simulink library "ExampleModel_lib"  (Simulink 7.9)
settings: Solver=ode45  StartTime=0.0  StopTime=10.0  RelTol=1e-3
libraries: powerlib x11, powerlib_extras x4, ExampleModel_lib x1
settings Model: RequirementInfo="{}  %GIDa_6317c1c3_1285_46a1_a401_c249d430af69"  Creator=jde1  LastModifiedBy=jde1

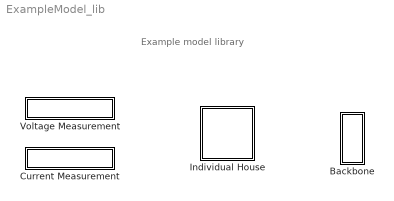
== system ExampleModel_lib ==
  note: Example model library
  Backbone : Subsystem  mask{length=0.0465}
  Current Measurement : Subsystem  StopFcn=|
      | myname = getfullname(gcb);                                                                      
      | rto = get_param([myname '/RMS Display'], 'RuntimeObject');                                      
      | set_param(myname, 'MaskDisplay', ['color(''blue''); disp(' num2str(rto.InputPort(1).Data) ')']);
      mask Display:
      | port_label('lconn', 1, '+')
      | port_label('rconn', 1, '-')
      | color('blue')
      | disp('0')
  Individual House : Subsystem  mask{length=0.02}
      mask prompts: length "Length of service line"
      mask Display:
      | plot([20 30 40 20 20 40 40], [30 40 30 30 10 10 30])
      | port_label('LConn',1,'+')
      | port_label('RConn',1,'-')
  Voltage Measurement : Subsystem  StopFcn=|
      | myname = getfullname(gcb);                                                                      
      | rto = get_param([myname '/RMS Display'], 'RuntimeObject');                                      
      | set_param(myname, 'MaskDisplay', ['color(''blue''); disp(' num2str(rto.InputPort(1).Data) ')']);
      mask Display:
      | port_label('lconn', 1, '+')
      | port_label('rconn', 1, '-')
      | color('blue')
      | disp('0')

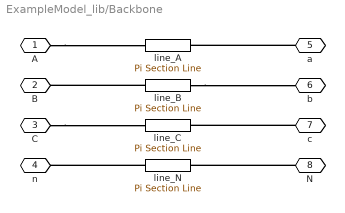
== system ExampleModel_lib/Backbone ==
  line_A : powerlib/Elements/Pi Section Line  LConnTagsString=__new0  RConnTagsString=__new0  Frequency=50  Resistance=0.497  Inductance=1.2032e-3  Capacitance=1e-9  Length=length  PiSections=1  Measurements=None
      settings: AttributesFormatString=\n
  line_B : powerlib/Elements/Pi Section Line  LConnTagsString=__new0  RConnTagsString=__new0  Frequency=50  Resistance=0.497  Inductance=1.2032e-3  Capacitance=1e-9  Length=length  PiSections=1  Measurements=None
      settings: AttributesFormatString=\n
  line_C : powerlib/Elements/Pi Section Line  LConnTagsString=__new0  RConnTagsString=__new0  Frequency=50  Resistance=0.497  Inductance=1.2032e-3  Capacitance=1e-9  Length=length  PiSections=1  Measurements=None
      settings: AttributesFormatString=\n
  line_N : powerlib/Elements/Pi Section Line  LConnTagsString=__new0  RConnTagsString=__new0  Frequency=50  Resistance=0.497  Inductance=1.2032e-3  Capacitance=1e-9  Length=length  PiSections=1  Measurements=None
      settings: AttributesFormatString=\n
  A : PMIOPort  Port=1  Side=Left
  B : PMIOPort  Port=2  Side=Left
  C : PMIOPort  Port=3  Side=Left
  n : PMIOPort  Port=4  Side=Left
  a : PMIOPort  Port=5  Side=Right
  b : PMIOPort  Port=6  Side=Right
  c : PMIOPort  Port=7  Side=Right
  N : PMIOPort  Port=8  Side=Right
  connections:
  line_N/RConn1 -- n/RConn1
  N/RConn1 -- line_N/LConn1
  a/RConn1 -- line_A/RConn1
  line_B/RConn1 -- b/RConn1
  c/RConn1 -- line_C/RConn1
  C/RConn1 -- line_C/LConn1
  line_B/LConn1 -- B/RConn1
  A/RConn1 -- line_A/LConn1

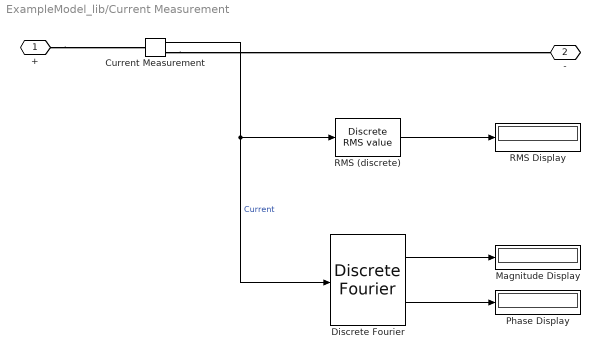
== system ExampleModel_lib/Current Measurement ==
  Current Measurement : powerlib/Measurements/Current Measurement  PhasorSimulation=off  OutputType=Complex  PSBequivalent=0
  Discrete Fourier : powerlib_extras/Discrete Measurements/Discrete  Fourier  Freq=50  n=1  Par_Init=[0 0]  Ts=0.001
  Magnitude Display : Display
  Phase Display : Display
  RMS (discrete) : powerlib_extras/Discrete Measurements/Discrete  RMS value  Freq=50  Mag_Init=0  Ts=0.001
  RMS Display : Display
  + : PMIOPort  Port=1  Side=Left
  - : PMIOPort  Port=2  Side=Right
  wires:
  RMS (discrete)/1 -> RMS Display/1
  Discrete Fourier/1 -> Magnitude Display/1
  Discrete Fourier/2 -> Phase Display/1
  Current Measurement/1 -> Discrete Fourier/1, RMS (discrete)/1  "Current"
  connections:
  +/RConn1 -- Current Measurement/LConn1
  Current Measurement/RConn1 -- -/RConn1

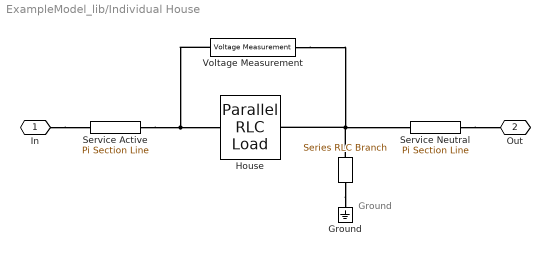
== system ExampleModel_lib/Individual House ==
  note: Ground
  " " : powerlib/Elements/Series RLC Branch  LConnTagsString=__new0  RConnTagsString=__new0  BranchType=R  Resistance=10  Inductance=1e-3  SetiL0=off  InitialCurrent=0  Capacitance=1e-6  Setx0=off  InitialVoltage=0  Measurements=None
  Ground : powerlib/Elements/Ground  LConnTagsString=a
  House : powerlib/Elements/Parallel RLC Load  LConnTagsString=a  RConnTagsString=__new0  NominalVoltage=230  NominalFrequency=50  ActivePower=500  InductivePower=1  CapacitivePower=1  Setx0=off  InitialVoltage=0  SetiL0=off  InitialCurrent=0  Measurements=None
      settings: AttributesFormatString=\n
  Service Active : powerlib/Elements/Pi Section Line  LConnTagsString=__new0  RConnTagsString=__new0  Frequency=50  Resistance=2.33  Inductance=2.833e-4  Capacitance=1e-9  Length=length  PiSections=1  Measurements=None
      settings: AttributesFormatString=\n
  Service Neutral : powerlib/Elements/Pi Section Line  LConnTagsString=__new0  RConnTagsString=__new0  Frequency=50  Resistance=2.33  Inductance=2.833e-4  Capacitance=1e-9  Length=length  PiSections=1  Measurements=None
      settings: AttributesFormatString=\n
  Voltage Measurement : ExampleModel_lib/Voltage Measurement  SystemSampleTime=-1
  In : PMIOPort  Port=1  Side=Left
  Out : PMIOPort  Port=2  Side=Right
  connections:
  Voltage Measurement/LConn1 -- House/LConn1 -- Service Active/RConn1
  " "/RConn1 -- Ground/LConn1
  " "/LConn1 -- House/RConn1 -- Voltage Measurement/RConn1 -- Service Neutral/LConn1
  In/RConn1 -- Service Active/LConn1
  Service Neutral/RConn1 -- Out/RConn1

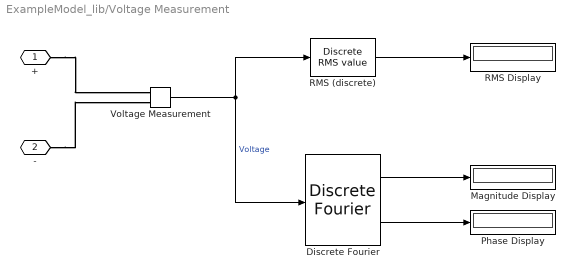
== system ExampleModel_lib/Voltage Measurement ==
  Discrete Fourier : powerlib_extras/Discrete Measurements/Discrete  Fourier  Freq=50  n=1  Par_Init=[0 0]  Ts=0.001
  Magnitude Display : Display
  Phase Display : Display
  RMS (discrete) : powerlib_extras/Discrete Measurements/Discrete  RMS value  Freq=50  Mag_Init=0  Ts=0.001
  RMS Display : Display
  Voltage Measurement : powerlib/Measurements/Voltage Measurement  PhasorSimulation=off  OutputType=Complex  PSBequivalent=0
  + : PMIOPort  Port=1  Side=Left
  - : PMIOPort  Port=2  Side=Right
  wires:
  Voltage Measurement/1 -> Discrete Fourier/1, RMS (discrete)/1  "Voltage"
  RMS (discrete)/1 -> RMS Display/1
  Discrete Fourier/1 -> Magnitude Display/1
  Discrete Fourier/2 -> Phase Display/1
  connections:
  +/RConn1 -- Voltage Measurement/LConn1
  -/RConn1 -- Voltage Measurement/LConn2
